simulink model "nonlinear"  (R2018b)
settings: Solver=VariableStepAuto  StartTime=0.0  StopTime=10.0  RelTol=1e-3
values from neighbouring files (symbols this model uses):
  j = 9.99*10^(-6)    (= 9.99e-06)    [nonlinearsim.m]    (also in stability.m)
  m = 0.11    [nonlinearsim.m]    (also in stability.m)
  N = -17.1874    [nonlinearsim.m]    (also in stability.m = inv(g))
  R = 0.015    [nonlinearsim.m]    (also in stability.m)
settings Model: Creator=hasti  LastModifiedBy=hasti

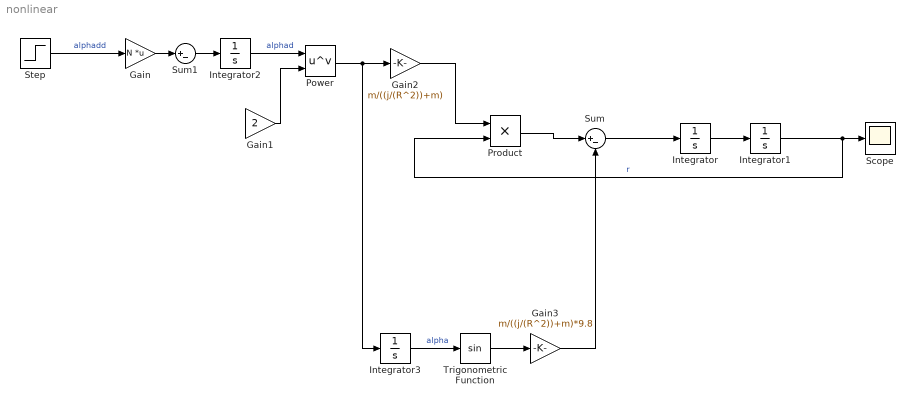
== system nonlinear ==
  Gain : Gain  Gain=N  Multiplication=Matrix(K*u)
  Gain1 : Gain  Gain=2
  Gain2 : Gain  Gain=m/((j/(R^2))+m)
  Gain3 : Gain  Gain=m/((j/(R^2))+m)*9.8
  Integrator{,1..3} (4 alike) : Integrator
  Power : Math  Operator=pow  SaturateOnIntegerOverflow=on
  Product : Product
  Scope : Scope
  Step : Step  Before=-5  SampleTime=0
  Sum : Sum  Inputs=|+-
  Sum1 : Sum  Inputs=|+-
  Trigonometric Function : Trigonometry
  wires:
  Sum/1 -> Integrator/1
  Integrator/1 -> Integrator1/1
  Integrator1/1 -> Product/2, Scope/1  "r"
  Step/1 -> Gain/1  "alphadd"
  Integrator2/1 -> Power/1  "alphad"
  Power/1 -> Integrator3/1, Gain2/1
  Gain1/1 -> Power/2
  Gain2/1 -> Product/1
  Product/1 -> Sum/1
  Integrator3/1 -> Trigonometric Function/1  "alpha"
  Trigonometric Function/1 -> Gain3/1
  Gain3/1 -> Sum/2
  Gain/1 -> Sum1/1
  Sum1/1 -> Integrator2/1
